simulink model "LR_3_var2"  (R2020b)
settings: Solver=VariableStepAuto  StartTime=0.0  StopTime=0.5  FixedStep=0.000001  RelTol=1e-3
settings Model: Creator=SIA  LastModifiedBy=SIA
settings SolverCC: ZeroCrossAlgorithm=Adaptive
settings DebuggingCC: IgnoredZcDiagnostic=none

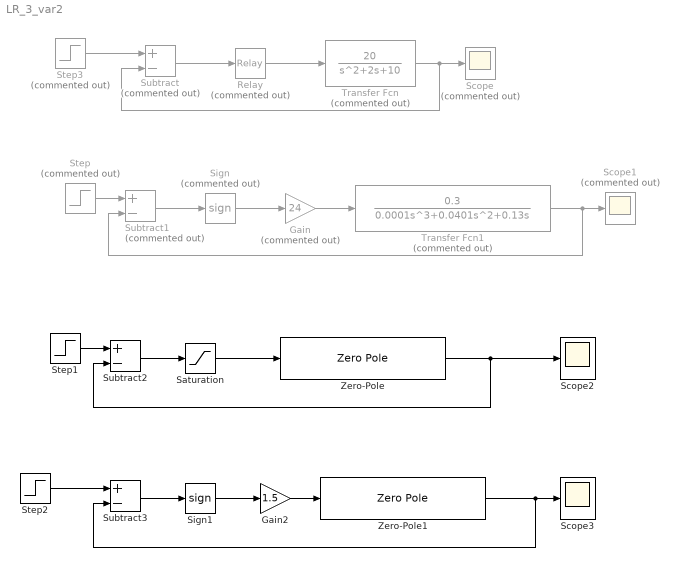
== system LR_3_var2 ==
  Gain : Gain  Commented=on  Gain=24
  Gain2 : Gain  Gain=1.5
  Relay : Relay  Commented=on  OnSwitchValue=0.5  OffSwitchValue=-0.5  OnOutputValue=0.5  OffOutputValue=-0.5
  Saturation : Saturate
  Scope : Scope  Commented=on
  Scope1 : Scope  Commented=on
  Scope2 : Scope
  Scope3 : Scope
  Sign : Signum  Commented=on
  Sign1 : Signum
  Step : Step  Commented=on  Time=0.01  Before=1  After=0  SampleTime=0
  Step1 : Step  Time=0.01  Before=1  After=0  SampleTime=0
  Step2 : Step  Time=0.01  Before=1  After=0  SampleTime=0
  Step3 : Step  Commented=on  Time=0.01  Before=1  After=0  SampleTime=0
  Subtract : Sum  Commented=on  Inputs=+-
  Subtract1 : Sum  Commented=on  Inputs=+-
  Subtract2 : Sum  Inputs=+-
  Subtract3 : Sum  Inputs=+-
  Transfer Fcn : TransferFcn  Commented=on  Numerator=[20]  Denominator=[1 2 10]
  Transfer Fcn1 : TransferFcn  Commented=on  Numerator=[0.3]  Denominator=[0.0001 0.0401 0.13 0]
  Zero-Pole : ZeroPole  Zeros=[-10 -10]  Poles=[-1 -1 -1]
  Zero-Pole1 : ZeroPole  Zeros=[-10 -10]  Poles=[-1 -1 -1]
  wires:
  Step3/1 -> Subtract/1
  Relay/1 -> Transfer Fcn/1
  Subtract/1 -> Relay/1
  Transfer Fcn/1 -> Scope/1, Subtract/2
  Subtract1/1 -> Sign/1
  Step/1 -> Subtract1/1
  Sign/1 -> Gain/1
  Transfer Fcn1/1 -> Scope1/1, Subtract1/2
  Gain/1 -> Transfer Fcn1/1
  Step1/1 -> Subtract2/1
  Zero-Pole/1 -> Scope2/1, Subtract2/2
  Subtract2/1 -> Saturation/1
  Saturation/1 -> Zero-Pole/1
  Subtract3/1 -> Sign1/1
  Sign1/1 -> Gain2/1
  Zero-Pole1/1 -> Scope3/1, Subtract3/2
  Gain2/1 -> Zero-Pole1/1
  Step2/1 -> Subtract3/1
